simulink library "BUMBLEBEE"  (R2024b)
settings: Solver=VariableStepAuto  StartTime=0.0  StopTime=10.0  RelTol=1e-3
settings Model: Creator=Mohammed Hany  LastModifiedBy=Mohammed Hany

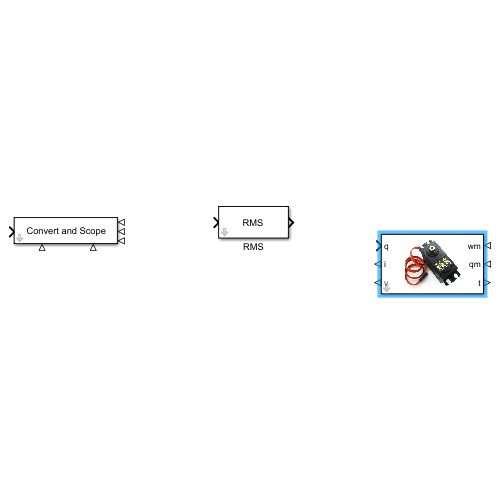
[thumbnail: Simulink's stored preview of the top-level diagram]
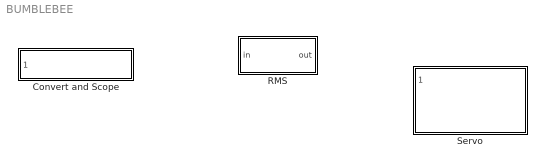
== system BUMBLEBEE ==
  Convert and Scope : Subsystem  ReferencedSubsystem=convert_and_scope
      settings: PortSchema="{\"entries\":[{\"content\":{\"sides\":[{\"content\":{\"connectorIds\":[\"LConn1\",\"LConn2\"]},\"type\":\"ConnectorPlacement.EquallySpacedRectSide\",\"uuid\":\"e9d3fa8a-a658-421c-a715-dee0f5d0277a\"},{\"content\":{\"side\":\"RIGHT\"},\"type\":\"ConnectorPlacement.EquallySpacedRectSide\",\"uuid\":\"8f4733ec-a2c9-48cc-bea1-8566252d8d79\"},{\"content\":{\"connectorIds\":[\"In1\"],\"side\":\"TOP\"},\"type\":\"ConnectorPlacement.EquallySpacedRectSide\",\"uuid\":\"ce7ba2ac-a2b1-42d2-bf3f-12c1e6573af0\"},{\"content\":{\"connectorIds\":[\"RConn1\",\"RConn2\",\"RConn3\"],\"side\":\"BOTTOM\"},\"type\":\"ConnectorPlacement.EquallySpacedRectSide\",\"uuid\":\"8390652c-32f7-42bc-a6e4-5fbde262c394\"}]},\"type\":\"ConnectorPlacement.EquallySpacedConnector\",\"uuid\":\"90170afb-acac-48c1-856c-2f07de9489fa\"}],\"packageUris\":[\"http://schema.mathworks.com/mf0/Connector/R2020b\"],\"version\":\"1.0\"}"
  RMS : Subsystem
      mask Display: disp('RMS');
  Servo : Subsystem  ReferencedSubsystem=Servo  J=0 cm^2*g  La=12e-6 H  P_rated=4.2 W  V_i_noload=6 V  V_rated=6 V  i_noload=0.05 A  w_max=99 rpm  w_rated=71.43 rpm  ratio=1

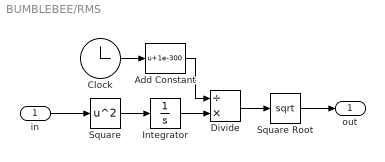
== system BUMBLEBEE/RMS ==
  in : Inport
  Add Constant : Bias  Bias=1e-300  SaturateOnIntegerOverflow=off
  Clock : Clock
  Divide : Product  Inputs=/*
  Integrator : Integrator
  Square : Math  Operator=square
  Square Root : Sqrt
  out : Outport
  wires:
  Square/1 -> Integrator/1
  Add Constant/1 -> Divide/1
  Integrator/1 -> Divide/2
  Clock/1 -> Add Constant/1
  in/1 -> Square/1
  Square Root/1 -> out/1
  Divide/1 -> Square Root/1
